simulink model "simEKFcamera"  (R2013a)
settings: Solver=ode3  StartTime=0.0  StopTime=t  FixedStep=0.001  RelTol=1e-3
undefined symbols (not defined in the file or in its folder): g, lengthBaseMiddle, magVecX, magVecY, magVecZ, sampleTime
settings Model: Creator=masters  LastModifiedBy=masters
settings SolverCC: AutoInsertRateTranBlk=on

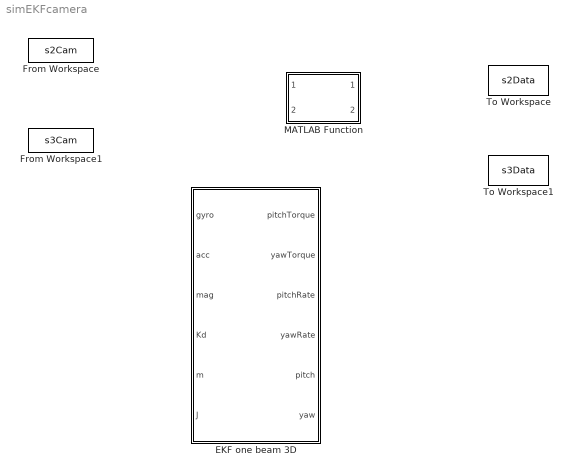
== system simEKFcamera ==
  "EKF one beam 3D " : MATLAB Function  TreatAsAtomicUnit=on  SystemSampleTime=sampleTime
  From Workspace : FromWorkspace  VariableName=s2Cam  SampleTime=0
  From Workspace1 : FromWorkspace  VariableName=s3Cam  SampleTime=0
  MATLAB Function : MATLAB Function  TreatAsAtomicUnit=on
  To Workspace : ToWorkspace  VariableName=s2Data  SampleTime=-1  SaveFormat=Timeseries
  To Workspace1 : ToWorkspace  VariableName=s3Data  SampleTime=-1  SaveFormat=Timeseries

== matlab function simEKFcamera/MATLAB Function ==
  data: s2Cam input; s2Data output; s3Cam input; s3Data output
function [s2Data,s3Data]= fcn(s2Cam,s3Cam)
%#codegen
persistent states;
persistent covP;
if isempty(states)
   states = [0 0 0 0 0 0]'; 
end

if isempty(covP)
    covP = [[1 0 0 0 0 0];
            [0 1 0 0 0 0];
            [0 0 1 0 0 0];
            [0 0 0 1 0 0];
            [0 0 0 0 1 0];
            [0 0 0 0 0 1]];
end

maxA=20;   
val=(maxA*J)^2*sampleTime^2;
Q = [[0     0      0              0               0        0];               
     [0     0      0              0               0        0];               
     [0     0      0              0               0        0];               
     [0     0      0              0               0        0];
     [0     0      0              0               0        0];
     [0     0      0              0               0        0]];      
 

R = [[0         0         0         0         0       0];      %accX
     [0         0         0         0         0       0];      %accZ
     [0         0         0         0         0       0];      %pitch rate
     [0         0         0         0         0       0];      %yaw rate
     [0         0         0         0         0       0];      %magX
     [0         0         0         0         0       0]]; %magY

I = [[1 0 0 0 0 0];
     [0 1 0 0 0 0];
     [0 0 1 0 0 0];
     [0 0 0 1 0 0];
     [0 0 0 0 1 0];
     [0 0 0 0 0 1]];
 
     
%PREDICT
s1x=states(1);
s1y=states(2);
s1z=states(3);
s2x=states(4);
s2y=states(5);
s2z=states(6);



states =[states(1) states(2) states(3) states(4) states(5) states(6)]'+sampleTime*[]';

s1x=states(1);
s1y=states(2);
s1z=states(3);
s2x=states(4);
s2y=states(5);
s2z=states(6);

%%TODO HERE 

F=I+sampleTime*[[0      0       0     0     0   0];
                [0      0       0     0     0   0];
                [0      0       0     0     0   0];
                [0      0       0     0     0   0];
                [0      0       0     0     0   0];
                [0      0       0     0     0   0]];
            
covP = (F)*(covP*(F')) + Q;

%UPDATE
H=[[1      0       0     0     0   0];%ax
   [0      1       0     0     0   0];%az
   [0      0       1     0     0   0];%gpitch
   [0      0       0     1     0   0];%gyaw 
   [0      0       0     0     1   0];%mx
   [0      0       0     0     0   1]];%my

K=covP*H'*inv(H*covP*H'+R);
z=[s2Cam(1) s2Cam(2) s2Cam(3) s3Cam(1) s3Cam(2) s3Cam(3)]';
y=states;
update=(z-y);
states=states+K*update;
covP=(I-K*H)*covP;
%output the date 

s1x=states(1);
s1y=states(2);
s1z=states(3);
s2x=states(4);
s2y=states(5);
s2z=states(6);

s2Date=[s1x s1y s1z]';
s3Date=[s2x s2y s2z]';

== matlab function simEKFcamera/EKF one beam 3D  ==
  data: gyro input; pitchTorque output; yawTorque output; acc input; mag input; sampleTime parameter; pitchRate output; lengthBaseMiddle parameter; Kd input; m input; g parameter; J input; yawRate output; pitch output; magVecX parameter; magVecY parameter; magVecZ parameter; yaw output
function [pitchTorque, yawTorque,pitchRate, yawRate, pitch,yaw]= fcn(gyro,acc,mag,sampleTime,lengthBaseMiddle,Kd,m,g,J,magVecX,magVecY,magVecZ)

persistent states;
persistent covP;
if isempty(states)
   states = [0 0 0 0 0 0]'; 
end

if isempty(covP)
    covP = [[1 0 0 0 0 0];
            [0 1 0 0 0 0];
            [0 0 1 0 0 0];
            [0 0 0 1 0 0];
            [0 0 0 0 1 0];
            [0 0 0 0 0 1]];
end

maxA=20;   
val=(maxA*J)^2*sampleTime^2;
Q = [[val   0      0              0               0        0];               
     [0     val    0              0               0        0];               
     [0     0      0.0000000008   0               0        0];               
     [0     0      0              0.000000008     0        0];
     [0     0      0              0               0        0];
     [0     0      0              0               0        0]];      
 

R = [[0.05      0         0         0         0       0];      %accX
     [0         0.5       0         0         0       0];      %accZ
     [0         0         0.00000006  0         0       0];      %pitch rate
     [0         0         0         0.000006       0       0];      %yaw rate
     [0         0         0         0         0.1  0];      %magX
     [0         0         0         0         0       0.1]]; %magY

I = [[1 0 0 0 0 0];
     [0 1 0 0 0 0];
     [0 0 1 0 0 0];
     [0 0 0 1 0 0];
     [0 0 0 0 1 0];
     [0 0 0 0 0 1]];
 
     
%PREDICT
appliedTpitchHat=states(1);
appliedTyawHat=states(2);
pitchRateHat=states(3);
yawRateHat=states(4);
pitchHat=states(5);
yawHat=states(6);

DTpitch=0;
DTyaw=0;

Dwpitch=(1/J)*(appliedTpitchHat-sign(pitchRateHat)*pitchRateHat^2*Kd*lengthBaseMiddle/2+lengthBaseMiddle*m*g*cos(pitchHat)/2);
Dwyaw=(1/J)*(appliedTyawHat-sign(yawRateHat)*yawRateHat^2*Kd*lengthBaseMiddle/2);

states =[states(1) states(2) states(3) states(4) states(5) states(6)]'+sampleTime*[DTpitch DTyaw Dwpitch Dwyaw pitchRateHat yawRateHat]';

appliedTpitchHat=states(1);
appliedTyawHat=states(2);
pitchRateHat=states(3);
yawRateHat=states(4);
pitchHat=states(5);
yawHat=states(6);

A=-pitchRateHat*Kd*lengthBaseMiddle/J;
B=-g*lengthBaseMiddle*m*sin(pitchHat)/(2*J);
C=-yawRateHat*Kd*lengthBaseMiddle/J;
F=I+sampleTime*[[0      0       0     0     0   0];
                [0      0       0     0     0   0];
                [1/J    0       A     0     B   0];
                [0      1/J     0     C     0   0];
                [0      0       1     0     0   0];
                [0      0       0     1     0   0]];
            
covP = (F)*(covP*(F')) + Q;

%UPDATE



ax=-pitchRateHat^2*lengthBaseMiddle+g*sin(pitchHat)-yawRateHat^2*lengthBaseMiddle;
az=Dwpitch*lengthBaseMiddle+g*cos(pitchHat);
mx=+cos(yawHat)*cos(pitchHat)*magVecX-sin(yawHat)*magVecY+cos(yawHat)*sin(pitchHat)*magVecZ;
my=sin(yawHat)*cos(pitchHat)*magVecX+cos(yawHat)*magVecY+sin(yawHat)*sin(pitchHat)*magVecZ;


A=-2*pitchRateHat*lengthBaseMiddle;
A1=-2*yawRateHat*lengthBaseMiddle;
B=g*cos(pitchHat);
C=-lengthBaseMiddle*pitchRateHat*Kd*lengthBaseMiddle/J;
D=-g*sin(pitchHat)-lengthBaseMiddle^2*m*g*sin(pitchHat)/(2*J);


E=-sin(pitchHat)*cos(yawHat)*magVecX+cos(pitchHat)*cos(yawHat)*magVecZ;
F=-cos(pitchHat)*sin(yawHat)*magVecX-cos(yawHat)*magVecY-sin(yawHat)*sin(pitchHat)*magVecZ;
G=-sin(pitchHat)*sin(yawHat)*magVecX+cos(pitchHat)*sin(yawHat)*magVecZ;
g=cos(yawHat)*cos(pitchHat)*magVecX-sin(yawHat)*magVecY+cos(yawHat)*sin(pitchHat)*magVecZ;

gyroYaw=yawRateHat/cos(pitchHat);

H=[[0                   0    A    A1                B                            0];%ax
   [lengthBaseMiddle/J  0    C    0                D                            0];%az
   [0                   0    1    0                0                            0];%gpitch
   [0                   0    0    1/cos(pitchHat)  sin(pitchHat)*yawRateHat/((cos(pitchHat))^2)    0];%gyaw 
   [0                   0    0    0                E                            F];%mx
   [0                   0    0    0                G                            g]];%my

K=covP*H'*inv(H*covP*H'+R);
z=[acc(2) acc(4) gyro(3) gyro(4) mag(2) mag(3)]';
y=[ax az states(3) gyroYaw mx my]';
update=(z-y);
states=states+K*update;
covP=(I-K*H)*covP;
%output the date 

pitchTorque=states(1);
yawTorque=states(2);
pitchRate=states(3);
yawRate=states(4);
pitch=states(5);
yaw=states(6);
